simulink model "TwoTankModel"  (R2025b)
settings: Solver=VariableStepAuto  StartTime=0.0  StopTime=3000  RelTol=1e-3

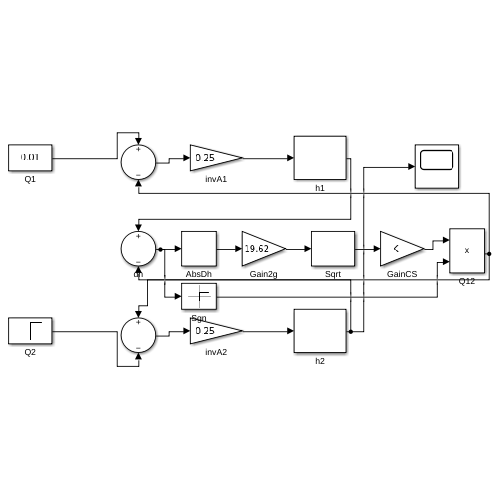
[thumbnail: Simulink's stored preview of the top-level diagram]
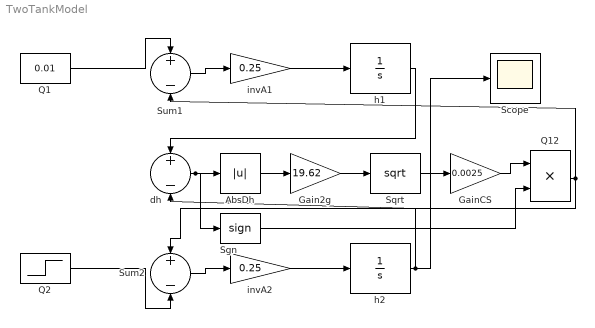
== system TwoTankModel ==
  AbsDh : Abs  SaturateOnIntegerOverflow=off
  Gain2g : Gain  Gain=19.62
  GainCS : Gain  Gain=0.0025
  Q1 : Constant  Value=0.01
  Q12 : Product
  Q2 : Step  Time=500  Before=0.01  After=0.012  SampleTime=0
  Scope : Scope
  Sgn : Signum
  Sqrt : Math  Operator=sqrt
  Sum1 : Sum  Inputs=+-
  Sum2 : Sum  Inputs=+-
  dh : Sum  Inputs=+-
  h1 : Integrator  InitialCondition=1.631
  h2 : Integrator  InitialCondition=0.81549
  invA1 : Gain  Gain=0.25
  invA2 : Gain  Gain=0.25
  wires:
  Q1/1 -> Sum1/1
  Q12/1 -> Sum1/2, Sum2/1
  Sum1/1 -> invA1/1
  invA1/1 -> h1/1
  h1/1 -> dh/1
  h2/1 -> dh/2, Scope/1
  dh/1 -> AbsDh/1, Sgn/1
  AbsDh/1 -> Gain2g/1
  Gain2g/1 -> Sqrt/1
  Sqrt/1 -> GainCS/1
  GainCS/1 -> Q12/1
  Sgn/1 -> Q12/2
  Q2/1 -> Sum2/2
  Sum2/1 -> invA2/1
  invA2/1 -> h2/1
